simulink model "Total"  (R2018b)
settings: Solver=VariableStepAuto  StartTime=0.0  StopTime=Tsim  RelTol=1e-3
values from neighbouring files (symbols this model uses):
  Bits_per_Sample = 8    [SetParamsVCO.m]
  DACSampleTime = 1/20000000    (= 5e-08)    [SetParamsVCO.m]
  h = gaussdesign(bt,span,sps)    [SetParamsVCO.m]
  Preamble = [0; 1; 1; 0; 1; 1; 1; 0; 0; 1]    [SetParamsVCO.m]
  PreambleInterval = 2^PreambleIntervalBits-1    (= 15)    [SetParamsVCO.m]
  SampleTime = 1/(Fsample_audio*Bits_per_Sample)    (= 4e-06)    [SetParamsVCO.m]
  SampleTimeUpsampler = 1/(Fsample_audio*10*Upsample_Rate)    (= 4e-07)    [SetParamsVCO.m]
libraries: commutil2 x7, dspsigops x3, simulink x2, commsynccomp2 x2, commrandsrc3 x1, commchan3 x1, commsink2 x1, dspswit3 x1, dspstat3 x1
settings Model: Creator=jellebakker  LastModifiedBy=Olaf
settings DebuggingCC: LibraryContextMissingDiagnostic=none
settings SFSimCC: SimUseLocalCustomCode=off
settings RTWCC: RTWUseLocalCustomCode=off

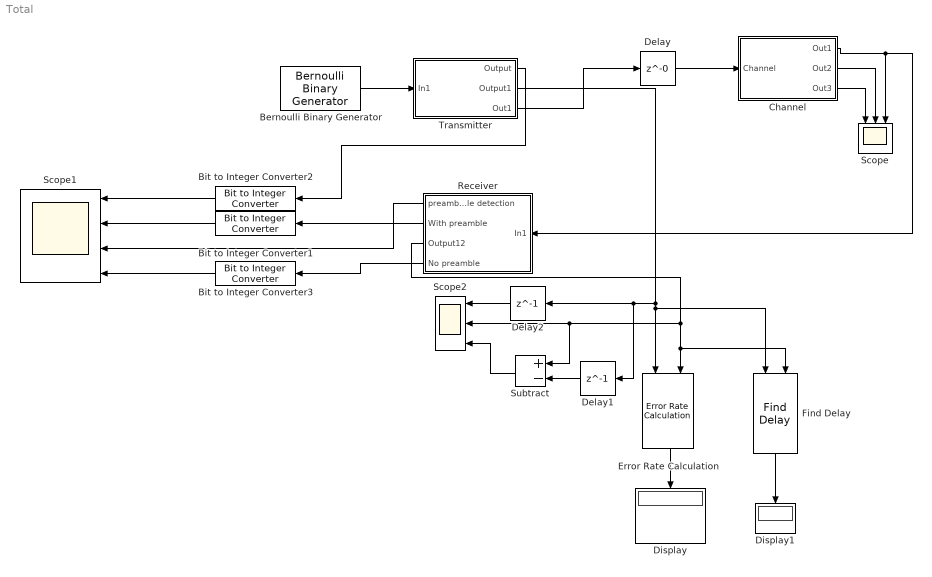
== system Total ==
  Bernoulli Binary Generator : commrandsrc3/Bernoulli Binary Generator  ProbabilityOfZero=0.5  SeedSource=Auto  Seed=0  SampleTime=SampleTime  SamplesPerFrame=Bits_per_Sample  OutputDataType=boolean  SimulateUsing=Interpreted execution
      settings: SourceProductName=Communications Toolbox
  Bit to Integer Converter1 : commutil2/Bit to Integer Converter  nbits=10  bitOrder=MSB first  signedOutputValues=Unsigned  outDtype=Inherit via internal rule  outDtypeSigned=Inherit via internal rule
      settings: SourceProductName=Communications Toolbox
  Bit to Integer Converter2 : commutil2/Bit to Integer Converter  nbits=10  bitOrder=MSB first  signedOutputValues=Unsigned  outDtype=Inherit via internal rule  outDtypeSigned=Inherit via internal rule
      settings: SourceProductName=Communications Toolbox
  Bit to Integer Converter3 : commutil2/Bit to Integer Converter  nbits=10  bitOrder=MSB first  signedOutputValues=Unsigned  outDtype=Inherit via internal rule  outDtypeSigned=Inherit via internal rule
      settings: SourceProductName=Communications Toolbox
  Channel : Subsystem
  Delay : Delay  DelayLength=0  SampleTime=50e-11
  Delay1 : Delay  DelayLength=1
  Delay2 : Delay  DelayLength=1
  Display : Display
  Display1 : Display
  Error Rate Calculation : commsink2/Error Rate Calculation  N=1  st_delay=0  cp_mode=Entire frame  subframe=[]  PMode=Port  WsName=ErrorVec  RsMode2=off  stop=off  numErr=100  maxBits=1e6
      settings: SourceProductName=Communications Toolbox
  Find Delay : commutil2/Find Delay  corrLength=120  chgSigOP=off  stopUpdate=off  numConstDelay=3
      settings: SourceProductName=Communications System Toolbox  SourceProductBaseCode=CM
  Receiver : Subsystem
  Scope : Scope  NumInputPorts=3
  Scope1 : Scope  NumInputPorts=4
  Scope2 : Scope  NumInputPorts=3
  Subtract : Sum  Inputs=+-
  Transmitter : Subsystem
  wires:
  Bernoulli Binary Generator/1 -> Transmitter/1(In1)
  Bit to Integer Converter2/1 -> Scope1/1
  Bit to Integer Converter1/1 -> Scope1/2
  Transmitter/2(Output1) -> Error Rate Calculation/1, Find Delay/1, Delay2/1, Delay1/1
  Receiver/3(Output12) -> Find Delay/2, Error Rate Calculation/2, Scope2/2, Subtract/1
  Receiver/1(preamble detection) -> Scope1/3
  Receiver/4(No preamble) -> Bit to Integer Converter3/1
  Bit to Integer Converter3/1 -> Scope1/4
  Error Rate Calculation/1 -> Display/1
  Find Delay/1 -> Display1/1
  Transmitter/1(Output) -> Bit to Integer Converter2/1
  Receiver/2(With preamble) -> Bit to Integer Converter1/1
  Channel/2(Out2) -> Scope/2
  Channel/1(Out1) -> Receiver/1(In1), Scope/3
  Delay/1 -> Channel/1(Channel)
  Channel/3(Out3) -> Scope/1
  Transmitter/3(Out1) -> Delay/1
  Subtract/1 -> Scope2/3
  Delay1/1 -> Subtract/2
  Delay2/1 -> Scope2/1

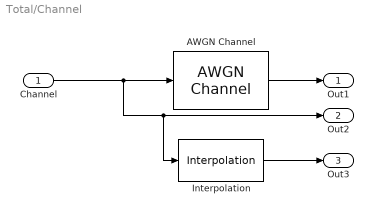
== system Total/Channel ==
  Channel : Inport
  AWGN Channel : commchan3/AWGN Channel  InputProcessing=Columns as channels (frame based)  seed=67  noiseMode="Signal to noise ratio  (SNR)"  EbNodB=10  EsNodB=10  SNRdB=15  bitsPerSym=1  Ps=1  Tsym=1  variance=1
      settings: SourceProductName=Communications Toolbox
  Interpolation : dspsigops/Interpolation  InterpSource=Specify via dialog  InterpPoints=[1.1 4.8 2.67 1.6 3.2]'  InterpMode=Linear  InterpL=3  InterpR=3  InterpAlpha=0.5  InvalidMode=Clip
      settings: SourceProductName=DSP System Toolbox  SourceProductBaseCode=DS
  Out1 : Outport
  Out2 : Outport  Port=2
  Out3 : Outport  Port=3
  wires:
  Channel/1 -> Interpolation/1, Out2/1, AWGN Channel/1
  AWGN Channel/1 -> Out1/1
  Interpolation/1 -> Out3/1

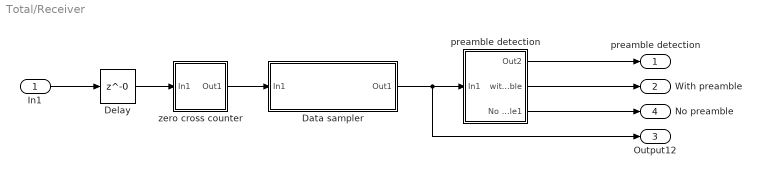
== system Total/Receiver ==
  In1 : Inport
  Data sampler : Subsystem
  Delay : Delay  DelayLength=0  SampleTime=50e-9
  "preamble detection " : Subsystem
  zero cross counter : Subsystem
  preamble detection : Outport
  With preamble : Outport  Port=2
  Output12 : Outport  Port=3
  No preamble : Outport  Port=4
  wires:
  In1/1 -> Delay/1
  "preamble detection "/2(with Preamble) -> With preamble/1
  "preamble detection "/1(Out2) -> preamble detection/1
  zero cross counter/1(Out1) -> Data sampler/1(In1)
  Data sampler/1(Out1) -> Output12/1, "preamble detection "/1(In1)
  "preamble detection "/3(No Preamble1) -> No preamble/1
  Delay/1 -> zero cross counter/1(In1)

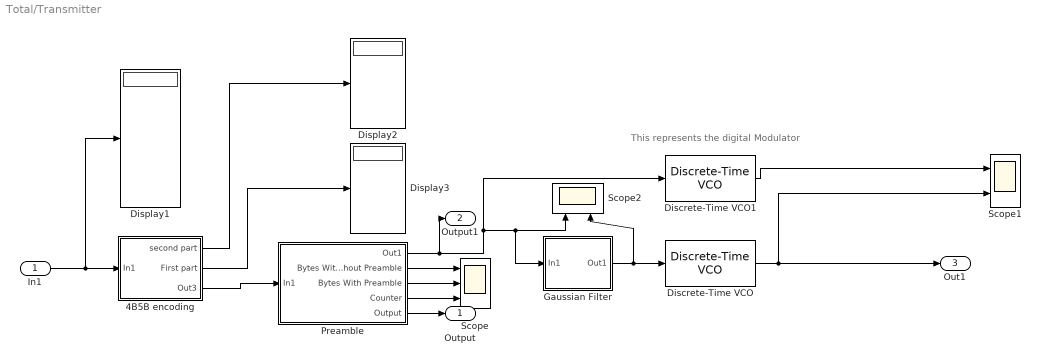
== system Total/Transmitter ==
  note: This represents the digital Modulator
  In1 : Inport
  4B5B encoding : Subsystem
  Discrete-Time VCO : commsynccomp2/Discrete-Time VCO  Ac=1  Fc=Quiescetf  Kc=InputSensitivity  Ph=0  ts=DACSampleTime
      settings: SourceProductName=Communications Toolbox  SourceProductBaseCode=CM
  Discrete-Time VCO1 : commsynccomp2/Discrete-Time VCO  Ac=1  Fc=Quiescetf  Kc=InputSensitivity  Ph=0  ts=DACSampleTime
      settings: SourceProductName=Communications Toolbox  SourceProductBaseCode=CM
  Display1 : Display
  Display2 : Display
  Display3 : Display
  Gaussian Filter : Subsystem
  Preamble : Subsystem
  Scope : Scope  NumInputPorts=3
  Scope1 : Scope  NumInputPorts=2
  Scope2 : Scope  NumInputPorts=2
  Output : Outport
  Output1 : Outport  Port=2
  Out1 : Outport  Port=3
  wires:
  Discrete-Time VCO/1 -> Out1/1, Scope1/2
  Gaussian Filter/1(Out1) -> Scope2/2, Discrete-Time VCO/1
  Discrete-Time VCO1/1 -> Scope1/1
  Preamble/2(Bytes Without Preamble) -> Scope/1
  In1/1 -> 4B5B encoding/1(In1), Display1/1
  Preamble/3(Bytes With Preamble) -> Scope/2
  4B5B encoding/1(second part) -> Display2/1
  Preamble/1(Out1) -> Output1/1, Gaussian Filter/1(In1), Scope2/1, Discrete-Time VCO1/1
  Preamble/4(Counter) -> Scope/3
  4B5B encoding/2(First part) -> Display3/1
  4B5B encoding/3(Out3) -> Preamble/1(In1)
  Preamble/5(Output) -> Output/1

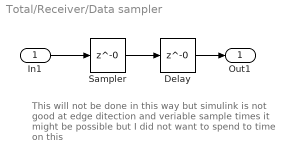
== system Total/Receiver/Data sampler ==
  note: This will not be done in this way but simulink is not
      | good at edge ditection and veriable sample times
      | it might be possible but I did not want to spend to
      | time on this
  In1 : Inport
  Delay : Delay  DelayLength=0  SampleTime=SampleTime*Bits_per_Sample/10
  Sampler : Delay  DelayLength=0  SampleTime=DACSampleTime/2
  Out1 : Outport
  wires:
  In1/1 -> Sampler/1
  Sampler/1 -> Delay/1
  Delay/1 -> Out1/1

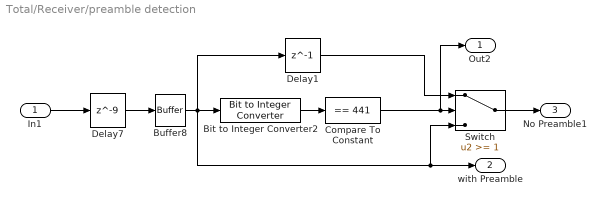
== system Total/Receiver/preamble detection  ==
  In1 : Inport
  Bit to Integer Converter2 : commutil2/Bit to Integer Converter  nbits=10  bitOrder=MSB first  signedOutputValues=Unsigned  outDtype=Inherit via internal rule  outDtypeSigned=Inherit via internal rule
      settings: SourceProductName=Communications Toolbox
  Buffer8 : Buffer  N=10  OutputFrames=off
  Compare To Constant : simulink/Logic and Bit Operations/Compare To Constant  relop===  const=441  OutDataTypeStr=boolean
  Delay1 : Delay  DelayLength=1
  Delay7 : Delay  DelayLength=9
  Switch : Switch  Threshold=1
  Out2 : Outport
  with Preamble : Outport  Port=2
  No Preamble1 : Outport  Port=3
  wires:
  Delay7/1 -> Buffer8/1
  In1/1 -> Delay7/1
  Compare To Constant/1 -> Switch/2, Out2/1
  Buffer8/1 -> Delay1/1, Bit to Integer Converter2/1, Switch/3, with Preamble/1
  Bit to Integer Converter2/1 -> Compare To Constant/1
  Delay1/1 -> Switch/1
  Switch/1 -> No Preamble1/1

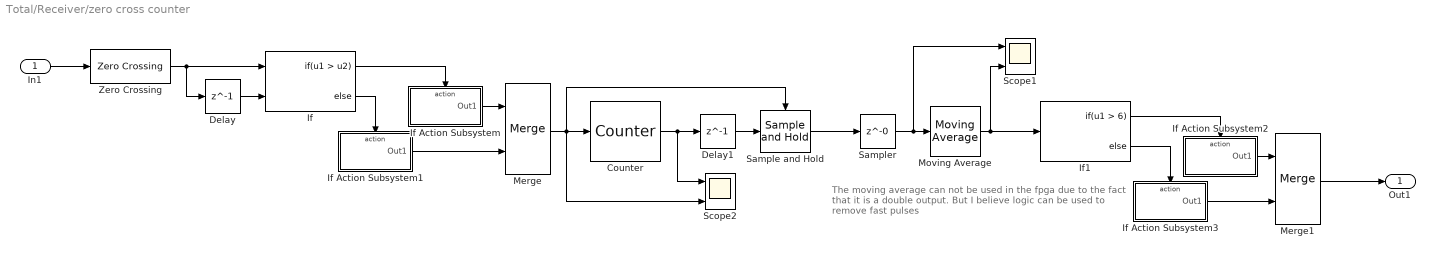
== system Total/Receiver/zero cross counter ==
  note: The moving average can not be used in the fpga due to the
      | fact that it is a double output. But I believe logic can be used
      | to remove fast pulses
  In1 : Inport
  Counter : dspswit3/Counter  Direction=Up  CountEvent=Free running  CounterSize=User defined  MaxCount=50000  InitialCount=0  Output=Count  HitValue=32  ResetInput=on  SamplesPerFrame=1  Ts=DACSampleTime  CntDtype=double  HitDtype=Logical
  Delay : Delay  DelayLength=1
  Delay1 : Delay  DelayLength=1  SampleTime=DACSampleTime/2
  If : If  NumInputs=2  IfExpression=u1 > u2
  If Action Subsystem : Subsystem  TreatAsAtomicUnit=on
  If Action Subsystem1 : Subsystem  TreatAsAtomicUnit=on
  If Action Subsystem2 : Subsystem  TreatAsAtomicUnit=on
  If Action Subsystem3 : Subsystem  TreatAsAtomicUnit=on
  If1 : If  IfExpression=u1 > 6
  Merge : Merge
  Merge1 : Merge
  Moving Average : dspstat3/Moving Average  Method=Sliding window  ForgettingFactorPort=off  SpecifyWindowLength=on  WindowLength=16  ForgettingFactor=0.9  SimulateUsing=Code generation
  Sample and Hold : dspsigops/Sample and Hold  trig=Rising edge  initCond=0  latchinput=off
  Sampler : Delay  DelayLength=0  SampleTime=DACSampleTime/2
  Scope1 : Scope  NumInputPorts=2
  Scope2 : Scope  NumInputPorts=2
  Zero Crossing : dspsigops/Zero Crossing
      settings: SourceProductName=DSP System Toolbox  SourceProductBaseCode=DS
  Out1 : Outport
  wires:
  Counter/1 -> Delay1/1, Scope2/1
  Merge/1 -> Sample and Hold/Trigger, Counter/1, Scope2/2
  Zero Crossing/1 -> Delay/1, If/1
  Moving Average/1 -> If1/1, Scope1/2
  Delay1/1 -> Sample and Hold/1
  Sampler/1 -> Scope1/1, Moving Average/1
  In1/1 -> Zero Crossing/1
  If/1 -> If Action Subsystem/Action
  Sample and Hold/1 -> Sampler/1
  If/2 -> If Action Subsystem1/Action
  If Action Subsystem1/1(Out1) -> Merge/2
  Delay/1 -> If/2
  If Action Subsystem/1(Out1) -> Merge/1
  If Action Subsystem2/1(Out1) -> Merge1/1
  If1/1 -> If Action Subsystem2/Action
  If Action Subsystem3/1(Out1) -> Merge1/2
  If1/2 -> If Action Subsystem3/Action
  Merge1/1 -> Out1/1

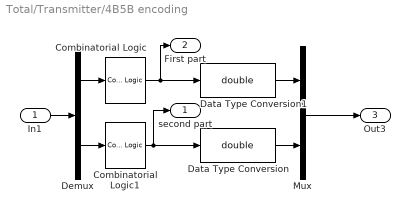
== system Total/Transmitter/4B5B encoding ==
  In1 : Inport
  Combinatorial Logic : CombinatorialLogic  TruthTable=[1 1 1 1 0;0 1 0 0 1;1 0 1 0 0;1 0 1 0 1;0 1 0 1 0;0 1 0 1 1;0 1 1 1 0;0 1 1 1 1;1 0 0 1 0;1 0 0 1 1;1 0 1 1 0;1 0 1 1 1;1 1 0 1 0;1 1 0 1 1;1 1 1 0 0;1 1 1 0 1]
  Combinatorial Logic1 : CombinatorialLogic  TruthTable=[1 1 1 1 0;0 1 0 0 1;1 0 1 0 0;1 0 1 0 1;0 1 0 1 0;0 1 0 1 1;0 1 1 1 0;0 1 1 1 1;1 0 0 1 0;1 0 0 1 1;1 0 1 1 0;1 0 1 1 1;1 1 0 1 0;1 1 0 1 1;1 1 1 0 0;1 1 1 0 1]
  Data Type Conversion : DataTypeConversion  OutDataTypeStr=double
  Data Type Conversion1 : DataTypeConversion  OutDataTypeStr=double
  Demux : Demux  Outputs=2
  Mux : Mux  Inputs=2
  second part : Outport
  First part : Outport  Port=2
  Out3 : Outport  Port=3
  wires:
  In1/1 -> Demux/1
  Combinatorial Logic/1 -> Data Type Conversion1/1, First part/1
  Data Type Conversion/1 -> Mux/2
  Mux/1 -> Out3/1
  Data Type Conversion1/1 -> Mux/1
  Demux/2 -> Combinatorial Logic1/1
  Demux/1 -> Combinatorial Logic/1
  Combinatorial Logic1/1 -> Data Type Conversion/1, second part/1

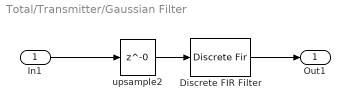
== system Total/Transmitter/Gaussian Filter ==
  In1 : Inport
  Discrete FIR Filter : DiscreteFir  Coefficients=h
  upsample2 : Delay  DelayLength=0  SampleTime=SampleTimeUpsampler
  Out1 : Outport
  wires:
  upsample2/1 -> Discrete FIR Filter/1
  Discrete FIR Filter/1 -> Out1/1
  In1/1 -> upsample2/1

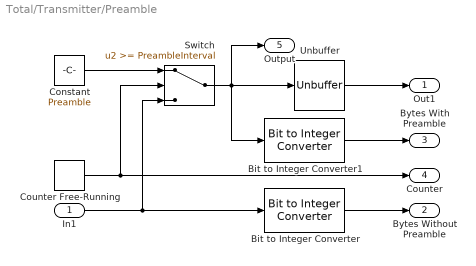
== system Total/Transmitter/Preamble ==
  In1 : Inport
  Bit to Integer Converter : commutil2/Bit to Integer Converter  nbits=10  bitOrder=MSB first  signedOutputValues=Unsigned  outDtype=Inherit via internal rule  outDtypeSigned=Inherit via internal rule
      settings: SourceProductName=Communications Toolbox
  Bit to Integer Converter1 : commutil2/Bit to Integer Converter  nbits=10  bitOrder=MSB first  signedOutputValues=Unsigned  outDtype=Inherit via internal rule  outDtypeSigned=Inherit via internal rule
      settings: SourceProductName=Communications Toolbox
  Constant : Constant  Value=Preamble  SampleTime=SampleTime*Bits_per_Sample
  Counter Free-Running : simulink/Sources/Counter Free-Running  NumBits=PreambleIntervalBits  tsamp=SampleTime*Bits_per_Sample
  Switch : Switch  Threshold=PreambleInterval
  Unbuffer : Unbuffer
  Out1 : Outport
  Bytes Without Preamble : Outport  Port=2
  Bytes With Preamble : Outport  Port=3
  Counter : Outport  Port=4
  Output : Outport  Port=5
  wires:
  Constant/1 -> Switch/1
  Counter Free-Running/1 -> Switch/2, Counter/1
  Switch/1 -> Output/1, Bit to Integer Converter1/1, Unbuffer/1
  Unbuffer/1 -> Out1/1
  In1/1 -> Switch/3, Bit to Integer Converter/1
  Bit to Integer Converter/1 -> Bytes Without Preamble/1
  Bit to Integer Converter1/1 -> Bytes With Preamble/1

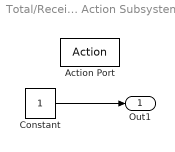
== system Total/Receiver/zero cross counter/If Action Subsystem ==
  Action Port : ActionPort  ActionType=then
  Constant : Constant
  Out1 : Outport
  wires:
  Constant/1 -> Out1/1

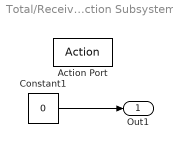
== system Total/Receiver/zero cross counter/If Action Subsystem1 ==
  Action Port : ActionPort  ActionType=else
  Constant1 : Constant  Value=0
  Out1 : Outport
  wires:
  Constant1/1 -> Out1/1

== system Total/Receiver/zero cross counter/If Action Subsystem2 ==
  Action Port : ActionPort  ActionType=then
  Constant : Constant  Value=0
  Out1 : Outport
  wires:
  Constant/1 -> Out1/1

== system Total/Receiver/zero cross counter/If Action Subsystem3 ==
  Action Port : ActionPort  ActionType=else
  Constant1 : Constant
  Out1 : Outport
  wires:
  Constant1/1 -> Out1/1
